simulink model "prova03"  (R2022b)
settings: Solver=VariableStepAuto  StartTime=0.0  StopTime=10.0  RelTol=1e-3
settings Model: Creator=giaco  LastModifiedBy=giaco

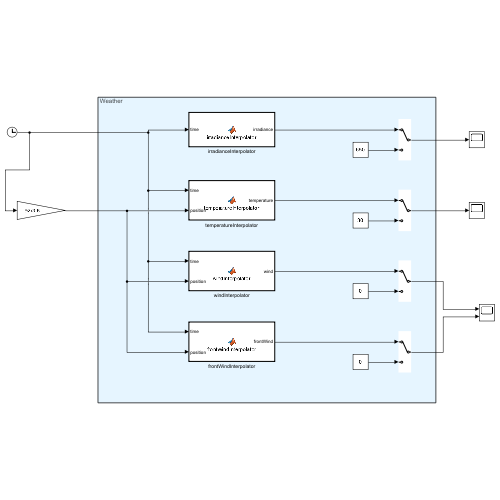
[thumbnail: Simulink's stored preview of the top-level diagram]
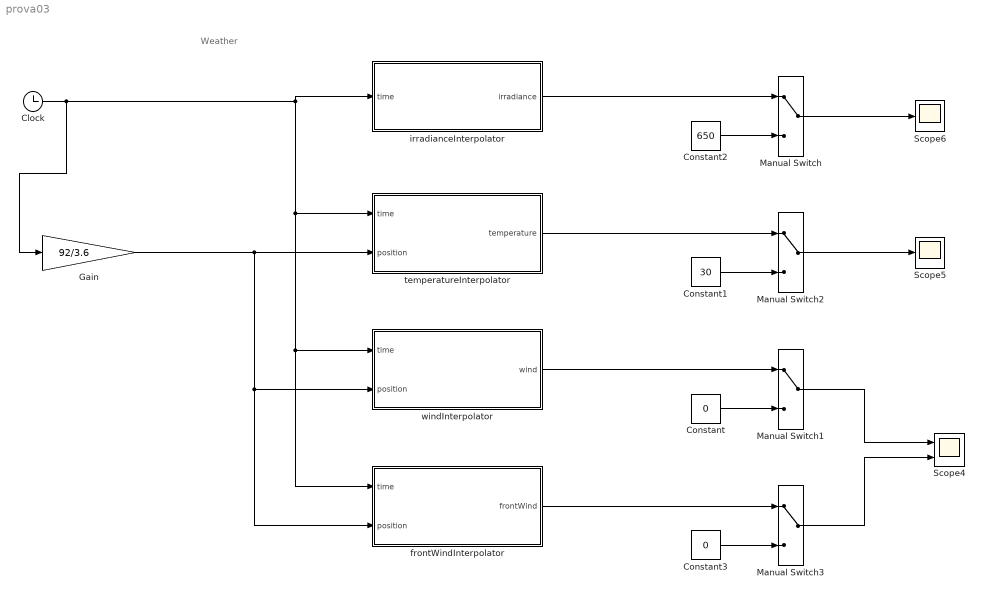
== system prova03 ==
  note: Weather
  Clock : Clock
  Constant : Constant  Value=0
  Constant1 : Constant  Value=30
  Constant2 : Constant  Value=650
  Constant3 : Constant  Value=0
  Gain : Gain  Gain=92/3.6
  Manual Switch{,1..3} (4 alike) : ManualSwitch
  Scope4 : Scope  NumInputPorts=2
  Scope5 : Scope
  Scope6 : Scope
  frontWindInterpolator : MATLAB Function  TreatAsAtomicUnit=on
  irradianceInterpolator : MATLAB Function  TreatAsAtomicUnit=on
  temperatureInterpolator : MATLAB Function  TreatAsAtomicUnit=on
  windInterpolator : MATLAB Function  TreatAsAtomicUnit=on
  wires:
  Gain/1 -> frontWindInterpolator/2(position), windInterpolator/2(position), temperatureInterpolator/2(position)
  Manual Switch1/1 -> Scope4/1
  windInterpolator/1(wind) -> Manual Switch1/1
  frontWindInterpolator/1(frontWind) -> Manual Switch3/1
  Constant/1 -> Manual Switch1/2
  Constant3/1 -> Manual Switch3/2
  Manual Switch2/1 -> Scope5/1
  Constant1/1 -> Manual Switch2/2
  Constant2/1 -> Manual Switch/2
  Manual Switch/1 -> Scope6/1
  Clock/1 -> irradianceInterpolator/1(time), frontWindInterpolator/1(time), windInterpolator/1(time), temperatureInterpolator/1(time), Gain/1
  Manual Switch3/1 -> Scope4/2
  irradianceInterpolator/1(irradiance) -> Manual Switch/1
  temperatureInterpolator/1(temperature) -> Manual Switch2/1

== matlab function prova03/temperatureInterpolator ==
  data: time input; position input; temperature output
function temperature = temperatureInterpolator(time, position)

coder.extrinsic('temperatureInterpolant02');

temperature = nan(1, 1);

temperature(1) = temperatureInterpolant02(time, position);

== matlab function prova03/irradianceInterpolator ==
  data: time input; irradiance output
function irradiance = irradianceInterpolator(time)

coder.extrinsic('irradianceInterpolant02');

irradiance = nan(1, 1);

irradiance(1) = irradianceInterpolant02(time);

== matlab function prova03/frontWindInterpolator ==
  data: time input; position input; frontWind output
function frontWind = frontWindInterpolator(time, position)

coder.extrinsic('frontWindInterpolant02');

frontWind = nan(1, 1);

frontWind(1) = frontWindInterpolant02(time, position);

== matlab function prova03/windInterpolator ==
  data: time input; position input; wind output
function wind = windInterpolator(time, position)

coder.extrinsic('windInterpolant02');

wind = nan(1, 1);

wind(1) = windInterpolant02(time, position);
